simulink model "pfb_fir_core"  (R2015b)
settings: Solver=VariableStepDiscrete  SolverMode=SingleTasking  StartTime=0.0  StopTime=2^(13-2+2)+100  RelTol=1e-3
undefined symbols (not defined in the file or in its folder): pfb_coeff_gen_calc
libraries: xbsIndex_r4 x684, casper_library_misc x40, casper_library_delays x24
(part 1 of 10)
settings Model: Creator=mdexter  LastModifiedBy=davidm
settings DataIOCC: SaveFormat=Array  SignalLoggingSaveFormat=ModelDataLogs
settings OptimizationCC: DefaultParameterBehavior=Inlined  ExpressionDepthLimit=2147483647
settings DebuggingCC: UnderspecifiedInitializationDetection=Classic  MergeDetectMultiDrivingBlocksExec=none  SolverPrmCheckMsg=warning  FcnCallInpInsideContextMsg=EnableAllAsWarning  StateNameClashWarn=warning
settings HardwareCC: ProdBitPerPointer=32  ProdLargestAtomicFloat=None  ProdIntDivRoundTo=Undefined  ProdEndianess=Unspecified  ProdWordSize=32  ProdHWDeviceType=32-bit Generic
settings GRTTargetCC: GeneratePreprocessorConditionals=Disable all
settings ConfigComp: CovModelRefEnable=Off

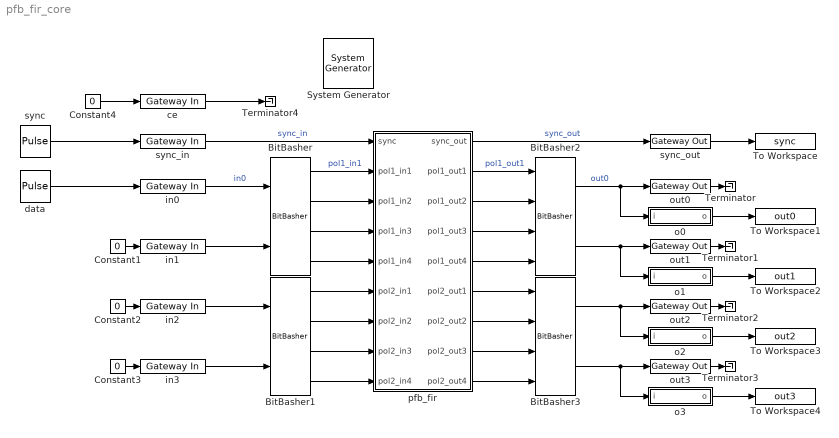
== system pfb_fir_core ==
  " System Generator" : xbsIndex_r4/ System Generator  Tag=genX  xilinxfamily=kintex7  part=xc7k160t  speed=-2  package=ffg676  synthesis_tool=XST  clock_wrapper=Clock Enables  directory=./pfb_fir_core  proj_type=Project Navigator  Synth_file=XST Defaults  Impl_file=ISE Defaults  testbench=off  simulink_period=1  sysclk_period=10  dcm_input_clock_period=10  incr_netlist=off  trim_vbits=Everywhere in SubSystem  dbl_ovrd=According to Block Masks  core_generation=According to Block Masks  run_coregen=off  deprecated_control=off  eval_field=0  block_type=sysgen
  BitBasher : xbsIndex_r4/BitBasher  bitexpr=|  display_expr=off  sr_1=1  arith_type1=Unsigned  bin_pt1=0  sr_2=2  arith_type2=Unsigned  bin_pt2=0  sr_3=3  arith_type3=Unsigned  bin_pt3=0  sr_4=4  arith_type4=Unsigned  bin_pt4=0  dbl_ovrd=off  block_type=bitbasher
      | <!DOCTYPE HTML PUBLIC "-//W3C//DTD HTML 4.0//EN" "http://www.w3.org/TR/REC-html40/strict.dtd">
      | <html><head><meta name="qrichtext" content="1" /><style type="text/css">
      | p, li { white-space: pre-wrap; }
      | </style></head><body style=" font-family:'Sans'; font-size:10pt; font-weight:400; font-style:normal;">
      | <p style=" margin-top:12px; margin-bottom:12px; margin-left:0px; margin-right:0px; -qt-block-indent:0; text-indent:0px;"><span style=" font-family:'MS Shell Dlg'; font-size:8pt;">o1={a[31:24], b[31:24]}<br />o2={a[23:16], b[23:16]}<br />o3={a[15:8], b[15:8]}<br />o4={a[7:0], b[7:0]}</span></p></body></html>
  BitBasher1 : xbsIndex_r4/BitBasher  bitexpr=|  display_expr=off  sr_1=1  arith_type1=Unsigned  bin_pt1=0  sr_2=2  arith_type2=Unsigned  bin_pt2=0  sr_3=3  arith_type3=Unsigned  bin_pt3=0  sr_4=4  arith_type4=Unsigned  bin_pt4=0  dbl_ovrd=off  block_type=bitbasher
      | <!DOCTYPE HTML PUBLIC "-//W3C//DTD HTML 4.0//EN" "http://www.w3.org/TR/REC-html40/strict.dtd">
      | <html><head><meta name="qrichtext" content="1" /><style type="text/css">
      | p, li { white-space: pre-wrap; }
      | </style></head><body style=" font-family:'Sans'; font-size:10pt; font-weight:400; font-style:normal;">
      | <p style=" margin-top:12px; margin-bottom:12px; margin-left:0px; margin-right:0px; -qt-block-indent:0; text-indent:0px;"><span style=" font-family:'MS Shell Dlg'; font-size:8pt;">o1={a[31:24], b[31:24]}<br />o2={a[23:16], b[23:16]}<br />o3={a[15:8], b[15:8]}<br />o4={a[7:0], b[7:0]}</span></p></body></html>
  BitBasher2 : xbsIndex_r4/BitBasher  bitexpr=|  display_expr=off  sr_1=1  arith_type1=Unsigned  bin_pt1=0  sr_2=2  arith_type2=Unsigned  bin_pt2=0  sr_3=3  arith_type3=Unsigned  bin_pt3=0  sr_4=4  arith_type4=Unsigned  bin_pt4=0  dbl_ovrd=off  block_type=bitbasher
      | <!DOCTYPE HTML PUBLIC "-//W3C//DTD HTML 4.0//EN" "http://www.w3.org/TR/REC-html40/strict.dtd">
      | <html><head><meta name="qrichtext" content="1" /><style type="text/css">
      | p, li { white-space: pre-wrap; }
      | </style></head><body style=" font-family:'Sans'; font-size:10pt; font-weight:400; font-style:normal;">
      | <p style=" margin-top:12px; margin-bottom:12px; margin-left:0px; margin-right:0px; -qt-block-indent:0; text-indent:0px;"><span style=" font-family:'MS Shell Dlg'; font-size:8pt;">a={i1[19:10], i2[19:10], i3[19:10], i4[19:10]}<br />b={i1[9:0], i2[9:0], i3[9:0], i4[9:0]}<br /></span></p></body></html>
  BitBasher3 : xbsIndex_r4/BitBasher  bitexpr=|  display_expr=off  sr_1=1  arith_type1=Unsigned  bin_pt1=0  sr_2=2  arith_type2=Unsigned  bin_pt2=0  sr_3=3  arith_type3=Unsigned  bin_pt3=0  sr_4=4  arith_type4=Unsigned  bin_pt4=0  dbl_ovrd=off  block_type=bitbasher
      | <!DOCTYPE HTML PUBLIC "-//W3C//DTD HTML 4.0//EN" "http://www.w3.org/TR/REC-html40/strict.dtd">
      | <html><head><meta name="qrichtext" content="1" /><style type="text/css">
      | p, li { white-space: pre-wrap; }
      | </style></head><body style=" font-family:'Sans'; font-size:10pt; font-weight:400; font-style:normal;">
      | <p style=" margin-top:12px; margin-bottom:12px; margin-left:0px; margin-right:0px; -qt-block-indent:0; text-indent:0px;"><span style=" font-family:'MS Shell Dlg'; font-size:8pt;">a={i1[19:10], i2[19:10], i3[19:10], i4[19:10]}<br />b={i1[9:0], i2[9:0], i3[9:0], i4[9:0]}<br /></span></p></body></html>
  Constant{1..4} (4 alike) : Constant  Value=0
  Terminator{,1..4} (5 alike) : Terminator
  To Workspace : ToWorkspace  VariableName=sync  SampleTime=-1
  To Workspace1 : ToWorkspace  VariableName=out0  SampleTime=-1
  To Workspace2 : ToWorkspace  VariableName=out1  SampleTime=-1
  To Workspace3 : ToWorkspace  VariableName=out2  SampleTime=-1
  To Workspace4 : ToWorkspace  VariableName=out3  SampleTime=-1
  ce : xbsIndex_r4/Gateway In  gui_display_data_type=Fixed-point  arith_type=Unsigned  n_bits=1  bin_pt=0  preci_type=Single  exp_width=8  frac_width=24  rows=1  columns=1  quantization="Round  (unbiased: +/- Inf)"  overflow=Saturate  period=1  UseAsADC=off  ADCChannel='1'  interface=None  automatic_assignment=on  address_offset=hex2dec('00')  intf_name=''  intf_description=''  default_value=0  timing_constraint=None  locs_specified=off  LOCs={}  io_standard={}  inherit_from_input=off  hdl_port=on  dbl_ovrd=off  block_type=gatewayin
  data : DiscretePulseGenerator  Amplitude=127*hex2dec('01010101')  Period=2^(13-2+2)+100  PulseWidth=2^(13-2)  PhaseDelay=3
  in{0..3} (4 alike) : xbsIndex_r4/Gateway In  gui_display_data_type=Fixed-point  arith_type=Unsigned  n_bits=32  bin_pt=0  preci_type=Single  exp_width=8  frac_width=24  rows=1  columns=1  quantization="Round  (unbiased: +/- Inf)"  overflow=Saturate  period=1  UseAsADC=off  ADCChannel='1'  interface=None  automatic_assignment=on  address_offset=hex2dec('00')  intf_name=''  intf_description=''  default_value=0  timing_constraint=None  locs_specified=off  LOCs={}  io_standard={}  inherit_from_input=off  hdl_port=on  dbl_ovrd=off  block_type=gatewayin
  o0 : Subsystem
  o1 : Subsystem
  o2 : Subsystem
  o3 : Subsystem
  out{0..3} (4 alike) : xbsIndex_r4/Gateway Out  inherit_from_input=off  hdl_port=on  rows=1  columns=1  UseAsDAC=off  DACChannel='1'  interface=None  automatic_assignment=on  address_offset=hex2dec('00')  intf_name=''  intf_description=''  timing_constraint=None  locs_specified=off  LOCs={}  io_standard={}  block_type=gatewayout
  pfb_fir : Subsystem  Tag=casper:pfb_fir  AncestorBlock=casper_library_pfbs/pfb_fir  mask(pfb_fir){PFBSize=13, TotalTaps=4, WindowType=hamming, n_inputs=2, MakeBiplex=on, BitWidthIn=8, BitWidthOut=10, CoeffBitWidth=18, CoeffDistMem=off, add_latency=1, mult_latency=3, bram_latency=3, fan_latency=1, quantization=Round  (unbiased: Even Values), fwidth=1, mult_spec=2, coeffs_share=on}
      mask prompts: PFBSize "Size of PFB: (2^? pnts)"; TotalTaps "Total Number of Taps:"; WindowType "Windowing Function:"; n_inputs "Number of Simultaneous Inputs: (2^?)"; MakeBiplex "Make Biplex?"; BitWidthIn "Input Bitwidth:"; BitWidthOut "Output Bitwidth:"; CoeffBitWidth "Coefficient Bitwidth:"; CoeffDistMem "Use Distributed Memory for Coeffs"; add_latency "Add Latency"; mult_latency "Mult Latency"; bram_latency "BRAM Latency"; fan_latency "Fanout Latency"; quantization "Quantization Behavior"; fwidth "Bin Width Scaling (normal=1)"; mult_spec "Multiplier specification (0=core, 1=embedded, 2=behavioural) (left=1st tap, or just one value)"; coeffs_share "Share coefficients between polarisations (use less BRAM)?"
      mask init:
      | pfb_fir_init(gcb, ...
      |     'PFBSize', PFBSize, ...
      |     'TotalTaps', TotalTaps, ...
      |     'WindowType', WindowType, ...
      |     'n_inputs', n_inputs, ...
      |     'MakeBiplex', MakeBiplex, ...
      |     'BitWidthIn', BitWidthIn, ...
      |     'BitWidthOut', BitWidthOut, ...
      |     'CoeffBitWidth', CoeffBitWidth, ...
      |     'CoeffDistMem', CoeffDistMem, ...
      |     'add_latency', add_latency, ...
      |     'mult_latency', mult_latency, ...
      |     'bram_latency', bram_latency, ...
      |     'fan_latency', fan_latency, ...
      |     'quantization', quantization, ...
      |     'fwidth', fwidth, ...
      |     'mult_spec', mult_spec, ...
      |     'coeffs_share', coeffs_share);
      settings: AttributesFormatString=|
      | taps=4, add_latency=1
      | max scale 0.596
      mask Help: eval('xlWeb(''http://casper.berkeley.edu/wiki/Pfb_fir'')')
      mask Callback TotalTaps:
      | %num_taps = eval(get_param(gcb, 'TotalTaps'));
      | %old_vec = eval(get_param(gcb, 'mult_spec'));
      | 
      | %vec = 2.*ones(1,num_taps);
      | %old_size = length(old_vec);
      | 
      | %if(old_size <= num_taps),
      | %   new_size = old_size;
      | %else,
      | %    new_size = num_taps;
      | %end
      | 
      | %for n = 1:new_size, vec(n) = old_vec(n); end
      | %set_param(gcb, 'mult_spec', mat2str(vec));
      mask TypeOptions WindowType: bartlett | barthannwin | blackman | blackmanharris | bohamwin | chebwin | flattopwin | gausswin | hamming | hann | kaiser | nuttallwin | parzenwin | rectwin | tukeywin | triang | userwindow
      mask TypeOptions quantization: Truncate | Round  (unbiased: +/- Inf) | Round  (unbiased: Even Values)
      mask Callback fwidth:
      | %num_taps = eval(get_param(gcb, 'TotalTaps'));
      | %old_vec = eval(get_param(gcb, 'mult_spec'));
      | 
      | %vec = 2.*ones(1,num_taps);
      | %old_size = length(old_vec);
      | 
      | %if(old_size <= num_taps),
      | %    new_size = old_size;
      | %else,
      | %    new_size = num_taps;
      | %end
      | 
      | %for n = 1:new_size, vec(n) = old_vec(n); end
      | %set_param(gcb, 'mult_spec', mat2str(vec));
      mask Callback mult_spec:
      | %num_taps = eval(get_param(gcb, 'TotalTaps'));
      | %old_vec = eval(get_param(gcb, 'mult_spec'));
      | 
      | %vec = 2.*ones(1,num_taps);
      | %old_size = length(old_vec);
      | 
      | %if(old_size <= num_taps),
      | %    new_size = old_size;
      | %else,
      | %    new_size = num_taps;
      | %end
      | 
      | %for n = 1:new_size, vec(n) = old_vec(n); end
      | %set_param(gcb, 'mult_spec', mat2str(vec));
  sync : DiscretePulseGenerator  Period=2^(13-2+2)+100  PhaseDelay=2
  sync_in : xbsIndex_r4/Gateway In  gui_display_data_type=Boolean  arith_type=Boolean  n_bits=16  bin_pt=14  preci_type=Single  exp_width=8  frac_width=24  rows=1  columns=1  quantization="Round  (unbiased: +/- Inf)"  overflow=Saturate  period=1  UseAsADC=off  ADCChannel='1'  interface=None  automatic_assignment=on  address_offset=hex2dec('00')  intf_name=''  intf_description=''  default_value=0  timing_constraint=None  locs_specified=off  LOCs={}  io_standard={}  inherit_from_input=off  hdl_port=on  dbl_ovrd=off  block_type=gatewayin
  sync_out : xbsIndex_r4/Gateway Out  inherit_from_input=off  hdl_port=on  rows=1  columns=1  UseAsDAC=off  DACChannel='1'  interface=None  automatic_assignment=on  address_offset=hex2dec('00')  intf_name=''  intf_description=''  timing_constraint=None  locs_specified=off  LOCs={}  io_standard={}  block_type=gatewayout
  wires:
  sync_in/1 -> pfb_fir/1(sync)  "sync_in"
  BitBasher/1 -> pfb_fir/2(pol1_in1)  "pol1_in1"
  BitBasher/2 -> pfb_fir/3(pol1_in2)
  BitBasher/3 -> pfb_fir/4(pol1_in3)
  BitBasher/4 -> pfb_fir/5(pol1_in4)
  BitBasher1/1 -> pfb_fir/6(pol2_in1)
  BitBasher1/2 -> pfb_fir/7(pol2_in2)
  BitBasher1/3 -> pfb_fir/8(pol2_in3)
  BitBasher1/4 -> pfb_fir/9(pol2_in4)
  in0/1 -> BitBasher/1  "in0"
  in1/1 -> BitBasher/2
  in2/1 -> BitBasher1/1
  in3/1 -> BitBasher1/2
  pfb_fir/1(sync_out) -> sync_out/1  "sync_out"
  Constant1/1 -> in1/1
  Constant2/1 -> in2/1
  Constant3/1 -> in3/1
  sync_out/1 -> To Workspace/1
  pfb_fir/2(pol1_out1) -> BitBasher2/1  "pol1_out1"
  pfb_fir/3(pol1_out2) -> BitBasher2/2
  pfb_fir/4(pol1_out3) -> BitBasher2/3
  pfb_fir/5(pol1_out4) -> BitBasher2/4
  pfb_fir/6(pol2_out1) -> BitBasher3/1
  pfb_fir/7(pol2_out2) -> BitBasher3/2
  pfb_fir/8(pol2_out3) -> BitBasher3/3
  pfb_fir/9(pol2_out4) -> BitBasher3/4
  BitBasher2/1 -> out0/1, o0/1(i)  "out0"
  BitBasher2/2 -> out1/1, o1/1(i)
  BitBasher3/1 -> out2/1, o2/1(i)
  BitBasher3/2 -> out3/1, o3/1(i)
  sync/1 -> sync_in/1
  data/1 -> in0/1
  o0/1(o) -> To Workspace1/1
  o1/1(o) -> To Workspace2/1
  o2/1(o) -> To Workspace3/1
  o3/1(o) -> To Workspace4/1
  out0/1 -> Terminator/1
  out1/1 -> Terminator1/1
  out2/1 -> Terminator2/1
  out3/1 -> Terminator3/1
  Constant4/1 -> ce/1
  ce/1 -> Terminator4/1

== system pfb_fir_core/o0 ==
  i : Inport
  BitBasher4 : xbsIndex_r4/BitBasher  bitexpr=|  display_expr=off  sr_1=1  arith_type1="Signed  (2's comp)"  bin_pt1=8  sr_2=2  arith_type2="Signed  (2's comp)"  bin_pt2=8  sr_3=3  arith_type3="Signed  (2's comp)"  bin_pt3=8  sr_4=4  arith_type4="Signed  (2's comp)"  bin_pt4=8  dbl_ovrd=off  block_type=bitbasher
      | <!DOCTYPE HTML PUBLIC "-//W3C//DTD HTML 4.0//EN" "http://www.w3.org/TR/REC-html40/strict.dtd">
      | <html><head><meta name="qrichtext" content="1" /><style type="text/css">
      | p, li { white-space: pre-wrap; }
      | </style></head><body style=" font-family:'Sans'; font-size:10pt; font-weight:400; font-style:normal;">
      | <p style=" margin-top:12px; margin-bottom:12px; margin-left:0px; margin-right:0px; -qt-block-indent:0; text-indent:0px;"><span style=" font-family:'MS Shell Dlg'; font-size:8pt;">o1={a[39:30]}<br />o2={a[29:20]}<br />o3={a[19:10]}<br />o4={a[9:0]}</span></p></body></html>
  Vector Concatenate : Concatenate  NumInputs=4
  o{1..4} (4 alike) : xbsIndex_r4/Gateway Out  inherit_from_input=off  hdl_port=off  rows=1  columns=1  UseAsDAC=off  DACChannel='1'  interface=None  automatic_assignment=on  address_offset=hex2dec('00')  intf_name=''  intf_description=''  timing_constraint=None  locs_specified=off  LOCs={}  io_standard={}  block_type=gatewayout
  o : Outport
  wires:
  BitBasher4/1 -> o1/1  "o1"
  BitBasher4/2 -> o2/1  "o2"
  BitBasher4/3 -> o3/1  "o3"
  BitBasher4/4 -> o4/1  "o4"
  o1/1 -> Vector Concatenate/1
  o2/1 -> Vector Concatenate/2
  o3/1 -> Vector Concatenate/3
  o4/1 -> Vector Concatenate/4
  i/1 -> BitBasher4/1
  Vector Concatenate/1 -> o/1

== system pfb_fir_core/o1 ==
  i : Inport
  BitBasher4 : xbsIndex_r4/BitBasher  bitexpr=|  display_expr=off  sr_1=1  arith_type1="Signed  (2's comp)"  bin_pt1=8  sr_2=2  arith_type2="Signed  (2's comp)"  bin_pt2=8  sr_3=3  arith_type3="Signed  (2's comp)"  bin_pt3=8  sr_4=4  arith_type4="Signed  (2's comp)"  bin_pt4=8  dbl_ovrd=off  block_type=bitbasher
      | <!DOCTYPE HTML PUBLIC "-//W3C//DTD HTML 4.0//EN" "http://www.w3.org/TR/REC-html40/strict.dtd">
      | <html><head><meta name="qrichtext" content="1" /><style type="text/css">
      | p, li { white-space: pre-wrap; }
      | </style></head><body style=" font-family:'Sans'; font-size:10pt; font-weight:400; font-style:normal;">
      | <p style=" margin-top:12px; margin-bottom:12px; margin-left:0px; margin-right:0px; -qt-block-indent:0; text-indent:0px;"><span style=" font-family:'MS Shell Dlg'; font-size:8pt;">o1={a[39:30]}<br />o2={a[29:20]}<br />o3={a[19:10]}<br />o4={a[9:0]}</span></p></body></html>
  Vector Concatenate : Concatenate  NumInputs=4
  o{1..4} (4 alike) : xbsIndex_r4/Gateway Out  inherit_from_input=off  hdl_port=off  rows=1  columns=1  UseAsDAC=off  DACChannel='1'  interface=None  automatic_assignment=on  address_offset=hex2dec('00')  intf_name=''  intf_description=''  timing_constraint=None  locs_specified=off  LOCs={}  io_standard={}  block_type=gatewayout
  o : Outport
  wires:
  Vector Concatenate/1 -> o/1
  i/1 -> BitBasher4/1
  o4/1 -> Vector Concatenate/4
  o3/1 -> Vector Concatenate/3
  o2/1 -> Vector Concatenate/2
  o1/1 -> Vector Concatenate/1
  BitBasher4/4 -> o4/1  "o4"
  BitBasher4/3 -> o3/1  "o3"
  BitBasher4/2 -> o2/1  "o2"
  BitBasher4/1 -> o1/1  "o1"

== system pfb_fir_core/o2 ==
  i : Inport
  BitBasher4 : xbsIndex_r4/BitBasher  bitexpr=|  display_expr=off  sr_1=1  arith_type1="Signed  (2's comp)"  bin_pt1=8  sr_2=2  arith_type2="Signed  (2's comp)"  bin_pt2=8  sr_3=3  arith_type3="Signed  (2's comp)"  bin_pt3=8  sr_4=4  arith_type4="Signed  (2's comp)"  bin_pt4=8  dbl_ovrd=off  block_type=bitbasher
      | <!DOCTYPE HTML PUBLIC "-//W3C//DTD HTML 4.0//EN" "http://www.w3.org/TR/REC-html40/strict.dtd">
      | <html><head><meta name="qrichtext" content="1" /><style type="text/css">
      | p, li { white-space: pre-wrap; }
      | </style></head><body style=" font-family:'Sans'; font-size:10pt; font-weight:400; font-style:normal;">
      | <p style=" margin-top:12px; margin-bottom:12px; margin-left:0px; margin-right:0px; -qt-block-indent:0; text-indent:0px;"><span style=" font-family:'MS Shell Dlg'; font-size:8pt;">o1={a[39:30]}<br />o2={a[29:20]}<br />o3={a[19:10]}<br />o4={a[9:0]}</span></p></body></html>
  Vector Concatenate : Concatenate  NumInputs=4
  o{1..4} (4 alike) : xbsIndex_r4/Gateway Out  inherit_from_input=off  hdl_port=off  rows=1  columns=1  UseAsDAC=off  DACChannel='1'  interface=None  automatic_assignment=on  address_offset=hex2dec('00')  intf_name=''  intf_description=''  timing_constraint=None  locs_specified=off  LOCs={}  io_standard={}  block_type=gatewayout
  o : Outport
  wires:
  BitBasher4/1 -> o1/1  "o1"
  BitBasher4/2 -> o2/1  "o2"
  BitBasher4/3 -> o3/1  "o3"
  BitBasher4/4 -> o4/1  "o4"
  o1/1 -> Vector Concatenate/1
  o2/1 -> Vector Concatenate/2
  o3/1 -> Vector Concatenate/3
  o4/1 -> Vector Concatenate/4
  i/1 -> BitBasher4/1
  Vector Concatenate/1 -> o/1

== system pfb_fir_core/o3 ==
  i : Inport
  BitBasher4 : xbsIndex_r4/BitBasher  bitexpr=|  display_expr=off  sr_1=1  arith_type1="Signed  (2's comp)"  bin_pt1=8  sr_2=2  arith_type2="Signed  (2's comp)"  bin_pt2=8  sr_3=3  arith_type3="Signed  (2's comp)"  bin_pt3=8  sr_4=4  arith_type4="Signed  (2's comp)"  bin_pt4=8  dbl_ovrd=off  block_type=bitbasher
      | <!DOCTYPE HTML PUBLIC "-//W3C//DTD HTML 4.0//EN" "http://www.w3.org/TR/REC-html40/strict.dtd">
      | <html><head><meta name="qrichtext" content="1" /><style type="text/css">
      | p, li { white-space: pre-wrap; }
      | </style></head><body style=" font-family:'Sans'; font-size:10pt; font-weight:400; font-style:normal;">
      | <p style=" margin-top:12px; margin-bottom:12px; margin-left:0px; margin-right:0px; -qt-block-indent:0; text-indent:0px;"><span style=" font-family:'MS Shell Dlg'; font-size:8pt;">o1={a[39:30]}<br />o2={a[29:20]}<br />o3={a[19:10]}<br />o4={a[9:0]}</span></p></body></html>
  Vector Concatenate : Concatenate  NumInputs=4
  o{1..4} (4 alike) : xbsIndex_r4/Gateway Out  inherit_from_input=off  hdl_port=off  rows=1  columns=1  UseAsDAC=off  DACChannel='1'  interface=None  automatic_assignment=on  address_offset=hex2dec('00')  intf_name=''  intf_description=''  timing_constraint=None  locs_specified=off  LOCs={}  io_standard={}  block_type=gatewayout
  o : Outport
  wires:
  Vector Concatenate/1 -> o/1
  i/1 -> BitBasher4/1
  o4/1 -> Vector Concatenate/4
  o3/1 -> Vector Concatenate/3
  o2/1 -> Vector Concatenate/2
  o1/1 -> Vector Concatenate/1
  BitBasher4/4 -> o4/1  "o4"
  BitBasher4/3 -> o3/1  "o3"
  BitBasher4/2 -> o2/1  "o2"
  BitBasher4/1 -> o1/1  "o1"
